simulink model "Motorized_Pendulum"  (R2020b)
settings: Solver=VariableStepAuto  StartTime=0.0  StopTime=6  RelTol=1e-6
undefined symbols (not defined in the file): g_n, Jm_n, Jp, K_2, K_3, Ka_fit, KcRa, Km_n, Kp, Kt, L_n, M_n, N_n, u_sel, v_ba
libraries: simulink x1, simulink_extras x1
settings Model: Creator=domin  LastModifiedBy=domin

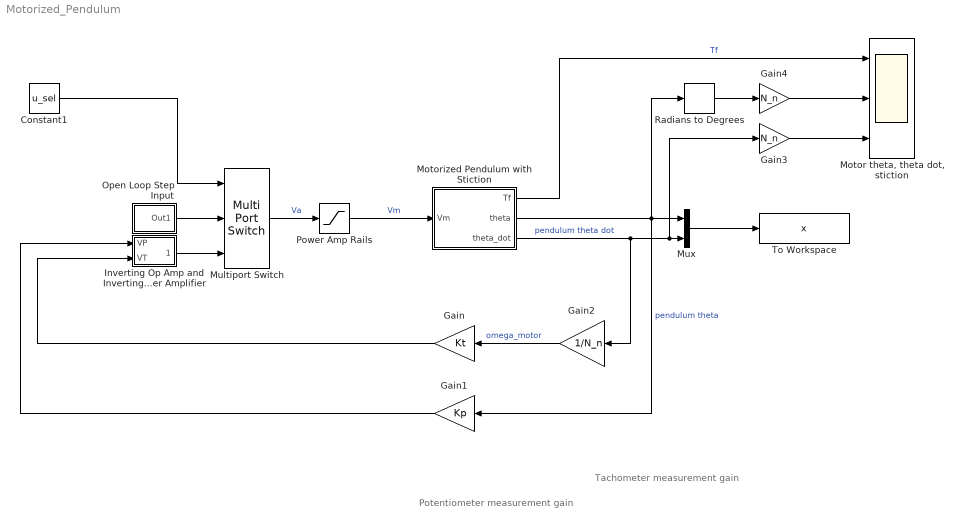
== system Motorized_Pendulum ==
  note: Potentiometer measurement gain
  note: Tachometer measurement gain
  Constant1 : Constant  Value=u_sel
  Gain : Gain  Gain=Kt
  Gain1 : Gain  Gain=Kp
  Gain2 : Gain  Gain=1/N_n
  Gain3 : Gain  Gain=N_n
  Gain4 : Gain  Gain=N_n
  Inverting Op Amp and Inverting Power Amplifier : Subsystem
  "Motor theta, theta dot, stiction" : Scope  NumInputPorts=3
  Motorized Pendulum with Stiction : Subsystem
  Multiport Switch : MultiPortSwitch  Inputs=2
  Mux : Mux  Inputs=2
  Open Loop Step Input : Subsystem
  Power Amp Rails : Saturate  UpperLimit=15  LowerLimit=-15
  Radians to Degrees : simulink_extras/Transformations/Radians to Degrees
  To Workspace : ToWorkspace  VariableName=x  SaveFormat=Timeseries  SampleTime=-1
  wires:
  Mux/1 -> To Workspace/1
  Radians to Degrees/1 -> Gain4/1
  Gain3/1 -> "Motor theta, theta dot, stiction"/3
  Gain4/1 -> "Motor theta, theta dot, stiction"/2
  Constant1/1 -> Multiport Switch/1
  Multiport Switch/1 -> Power Amp Rails/1  "Va"
  Motorized Pendulum with Stiction/2(theta) -> Gain1/1, Mux/1, Radians to Degrees/1  "pendulum theta"
  Motorized Pendulum with Stiction/3(theta_dot) -> Gain2/1, Mux/2, Gain3/1  "pendulum theta dot"
  Power Amp Rails/1 -> Motorized Pendulum with Stiction/1(Vm)  "Vm"
  Motorized Pendulum with Stiction/1(Tf) -> "Motor theta, theta dot, stiction"/1  "Tf"
  Open Loop Step Input/1(Out1) -> Multiport Switch/2
  Gain2/1 -> Gain/1  "omega_motor"
  Gain/1 -> Inverting Op Amp and Inverting Power Amplifier/2(VT)
  Inverting Op Amp and Inverting Power Amplifier/1(Out1) -> Multiport Switch/3
  Gain1/1 -> Inverting Op Amp and Inverting Power Amplifier/1(VP)

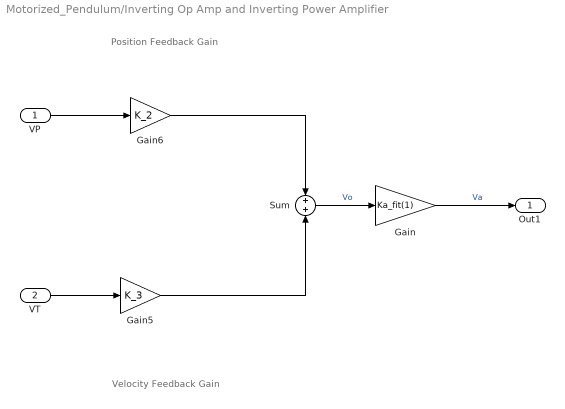
== system Motorized_Pendulum/Inverting Op Amp and Inverting Power Amplifier ==
  note: Position Feedback Gain
  note: Velocity Feedback Gain
  VP : Inport
  VT : Inport  Port=2
  Gain : Gain  Gain=Ka_fit(1)
  Gain5 : Gain  Gain=K_3
  Gain6 : Gain  Gain=K_2
  Sum : Sum
  Out1 : Outport
  wires:
  VT/1 -> Gain5/1
  VP/1 -> Gain6/1
  Gain6/1 -> Sum/1
  Gain5/1 -> Sum/2
  Sum/1 -> Gain/1  "Vo"
  Gain/1 -> Out1/1  "Va"

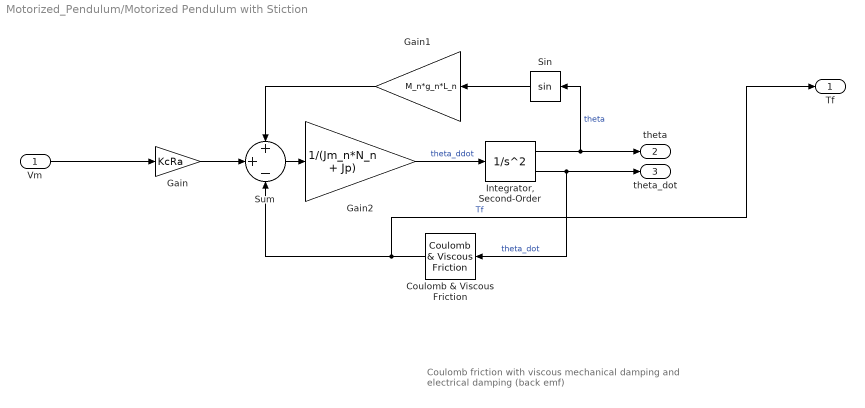
== system Motorized_Pendulum/Motorized Pendulum with Stiction ==
  note: Coulomb friction with viscous mechanical damping
      | and electrical damping (back emf)
  Vm : Inport
  Coulomb & Viscous Friction : simulink/Discontinuities/Coulomb & Viscous Friction  offset=T_ba  gain=N_n*KcRa/Km_n
  Gain : Gain  Gain=KcRa
  Gain1 : Gain  Gain=M_n*g_n*L_n
  Gain2 : Gain  Gain=1/(Jm_n*N_n + Jp)
  "Integrator, Second-Order" : SecondOrderIntegrator  WrapX=on
  Sin : Trigonometry
  Sum : Sum  Inputs=++-
  Tf : Outport
  theta : Outport  Port=2
  theta_dot : Outport  Port=3
  wires:
  Gain2/1 -> "Integrator, Second-Order"/1  "theta_ddot"
  Sin/1 -> Gain1/1
  "Integrator, Second-Order"/2 -> theta_dot/1, Coulomb & Viscous Friction/1  "theta_dot"
  Coulomb & Viscous Friction/1 -> Tf/1, Sum/3  "Tf"
  "Integrator, Second-Order"/1 -> theta/1, Sin/1  "theta"
  Gain1/1 -> Sum/1
  Sum/1 -> Gain2/1
  Vm/1 -> Gain/1
  Gain/1 -> Sum/2

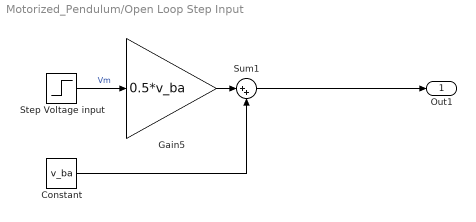
== system Motorized_Pendulum/Open Loop Step Input ==
  Constant : Constant  Value=v_ba
  Gain5 : Gain  Gain=0.5*v_ba
  Step Voltage input : Step  SampleTime=0
  Sum1 : Sum  Inputs=|++
  Out1 : Outport
  wires:
  Sum1/1 -> Out1/1
  Step Voltage input/1 -> Gain5/1  "Vm"
  Gain5/1 -> Sum1/1
  Constant/1 -> Sum1/2
